simulink library "Average"  (R2018b)
settings: Solver=ode45  StartTime=0.0  StopTime=10.0  RelTol=1e-3  EnableMultiTasking=on
settings Model: Creator=lena.frank  LastModifiedBy=drhf
settings DataIOCC: LimitDataPoints=on  SaveFormat=Array  SignalLoggingSaveFormat=ModelDataLogs
settings OptimizationCC: ExpressionDepthLimit=2147483647  LifeSpan=inf
settings DebuggingCC: UnderspecifiedInitializationDetection=Classic  MergeDetectMultiDrivingBlocksExec=none  SolverPrmCheckMsg=warning  FcnCallInpInsideContextMsg=warning  StateNameClashWarn=warning  SFUnexpectedBacktrackingDiag=warning  SFNoUnconditionalDefaultTransitionDiag=warning  SFExecutionAtInitializationDiag=none
settings HardwareCC: ProdBitPerPointer=32  ProdBitPerSizeT=32  ProdBitPerPtrDiffT=32  ProdLargestAtomicFloat=None  ProdIntDivRoundTo=Undefined  ProdEndianess=Unspecified  ProdWordSize=32  ProdHWDeviceType=32-bit Generic
settings ModelReferenceCC: PropagateSignalLabelsOutOfModel=off
settings SFSimCC: SimUseLocalCustomCode=off
settings RTWCC: RTWUseLocalCustomCode=off
settings CodeAppCC: StateflowObjectComments=on
settings GRTTargetCC: TargetLangStandard=C89/C90 (ANSI)  GeneratePreprocessorConditionals=Disable all  CombineOutputUpdateFcns=off  GRTInterface=on
settings ConfigComp: CovMetricSettings=dw  CovHtmlReporting=on  CovSaveCumulativeToWorkspaceVar=on  CovSaveSingleToWorkspaceVar=on  CovExternalEMLEnable=off

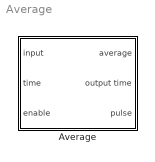
== system Average ==
  Average : Subsystem  mask{time_intervall=3600, offset_flag=off, enable_flag=off}
      mask prompts: time_intervall "Delta_t in s"; offset_flag "start calculating every full hour"; enable_flag "only calculate when enabled"
      mask help:
      | This block calculates the average of each input vector during a specified time Delta_t. During this time interval the output is held.
      | The output time is the time of the last average calculation. Every time the average is calculated again, a signal pulse of 1 is put out.
      | When the full hour flag is set, the calculation of the average is started every full hour once again.
      | When the enable flag is set, the functions calculates only while the enable signal is 1. When it is 0, the function repeats putting out the last output.
      mask init:
      | if time_intervall==0
      |     delta_t = 1;
      | else
      |     delta_t = time_intervall;
      | end
      mask Help: web(fullfile(path_carnot('help'),'Average.html'),'-helpbrowser')

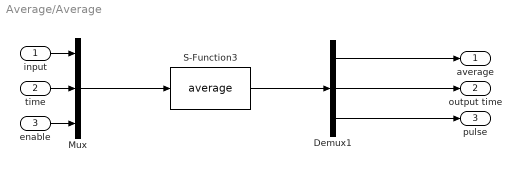
== system Average/Average ==
  input : Inport
  time : Inport  Port=2
  enable : Inport  Port=3
  Demux1 : Demux  Outputs=[-1 1 1]
  Mux : Mux  Inputs=3
  S-Function3 : S-Function  FunctionName=average  Parameters=delta_t offset_flag enable_flag  SFunctionDeploymentMode=off  EnableBusSupport=off  SFcnStateName=D_LAST_OUTPUT
      settings: SFcnIsStateOwnerBlock=on
  average : Outport
  output time : Outport  Port=2
  pulse : Outport  Port=3
  wires:
  Demux1/1 -> average/1
  Demux1/3 -> pulse/1
  time/1 -> Mux/2
  Demux1/2 -> output time/1
  S-Function3/1 -> Demux1/1
  input/1 -> Mux/1
  enable/1 -> Mux/3
  Mux/1 -> S-Function3/1
